simulink model "abs"  (R2023b)
settings: Solver=VariableStepAuto  StartTime=0.0  StopTime=25  RelTol=1e-3
undefined symbols (not defined in the file): g, I, m, muCoefficientOfFriction, R, Slip, v0
settings Model: Creator=Asus  LastModifiedBy=Asus

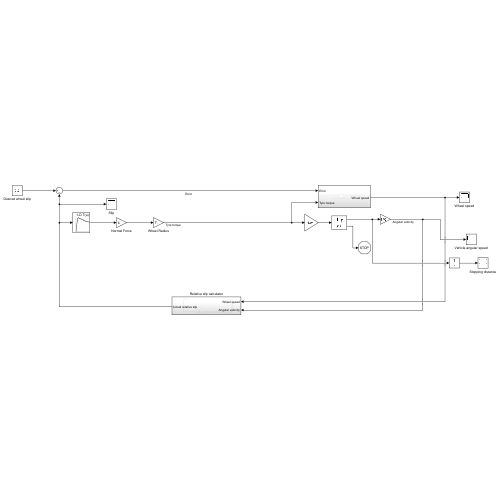
[thumbnail: Simulink's stored preview of the top-level diagram]
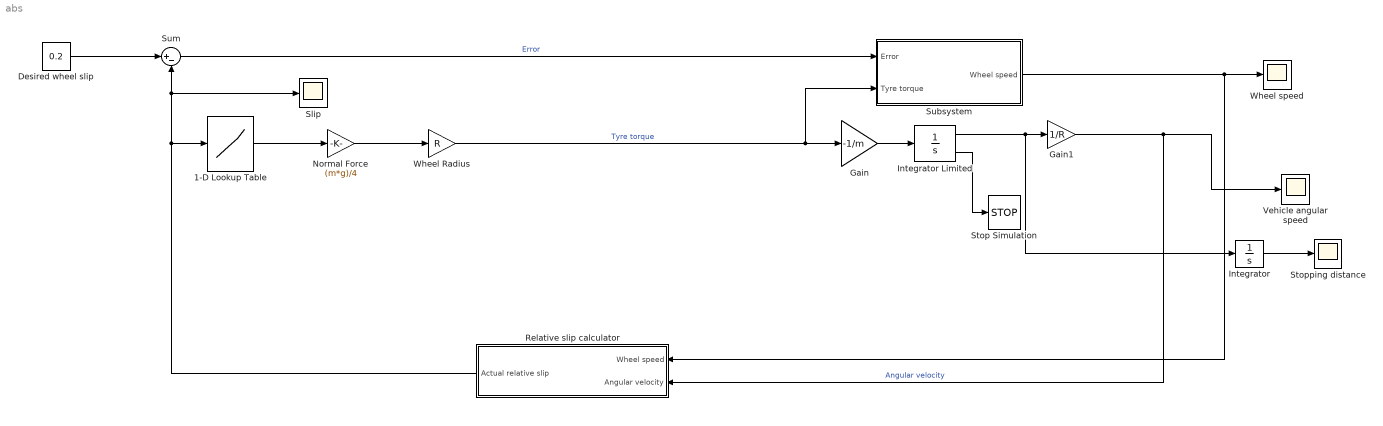
== system abs ==
  1-D Lookup Table : Lookup_n-D  NumberOfTableDimensions=1  BreakpointsForDimension1=muCoefficientOfFriction  Table=Slip  InternalRulePriority=Speed  RndMeth=Simplest
  Desired wheel slip : Constant  Value=0.2  SampleTime=-1
  Gain : Gain  Gain=-1/m
  Gain1 : Gain  Gain=1/R
  Integrator : Integrator
  Integrator Limited : Integrator  InitialCondition=v0  LimitOutput=on  UpperSaturationLimit=1000  LowerSaturationLimit=0  ShowSaturationPort=on
  Normal Force : Gain  Gain=(m*g)/4
  Relative slip calculator : Subsystem
  Slip : Scope
  Stop Simulation : Stop
  Stopping distance : Scope
  Subsystem : Subsystem
  Sum : Sum  Inputs=|+-
  Vehicle angular speed : Scope
  Wheel Radius : Gain  Gain=R
  Wheel speed : Scope
  wires:
  Desired wheel slip/1 -> Sum/1
  1-D Lookup Table/1 -> Normal Force/1
  Normal Force/1 -> Wheel Radius/1
  Sum/1 -> Subsystem/1(Error)  "Error"
  Wheel Radius/1 -> Gain/1, Subsystem/2(Tyre torque)  "Tyre torque"
  Subsystem/1(Wheel speed) -> Wheel speed/1, Relative slip calculator/1(Wheel speed)
  Gain/1 -> Integrator Limited/1
  Integrator Limited/2 -> Stop Simulation/1
  Integrator Limited/1 -> Integrator/1, Gain1/1
  Gain1/1 -> Relative slip calculator/2(Angular velocity), Vehicle angular speed/1  "Angular velocity"
  Integrator/1 -> Stopping distance/1
  Relative slip calculator/1(Actual relative slip) -> 1-D Lookup Table/1, Slip/1, Sum/2

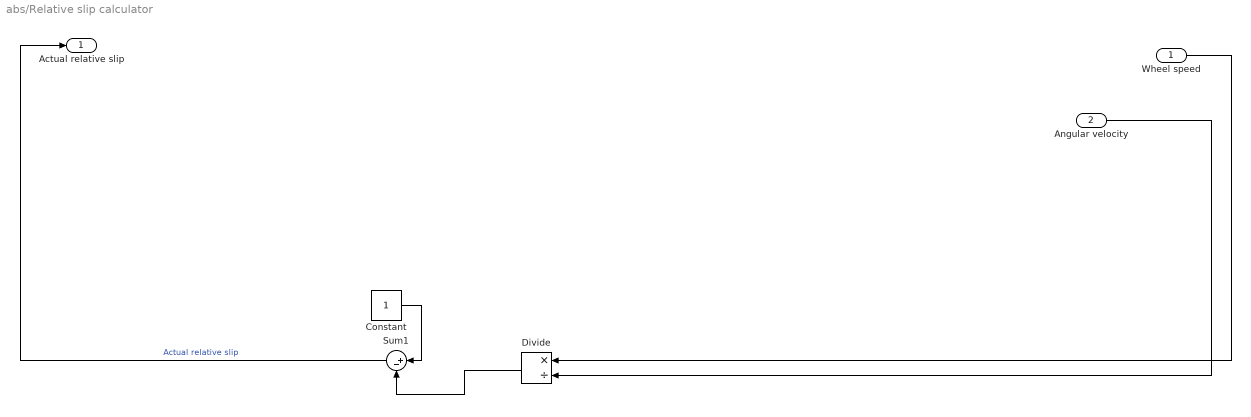
== system abs/Relative slip calculator ==
  Wheel speed : Inport
  Angular velocity : Inport  Port=2
  Constant : Constant
  Divide : Product  Inputs=*/
  Sum1 : Sum  Inputs=|+-
  Actual relative slip : Outport
  wires:
  Constant/1 -> Sum1/1
  Divide/1 -> Sum1/2
  Angular velocity/1 -> Divide/2
  Sum1/1 -> Actual relative slip/1  "Actual relative slip"
  Wheel speed/1 -> Divide/1

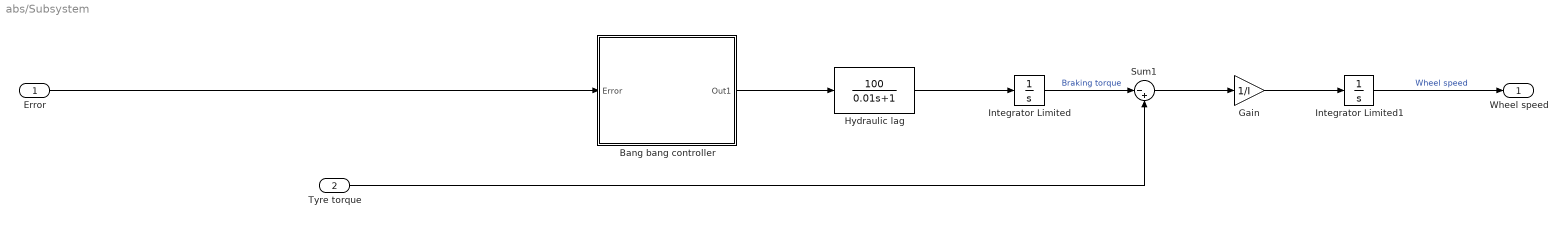
== system abs/Subsystem ==
  Error : Inport
  Tyre torque : Inport  Port=2
  Bang bang controller : Subsystem
  Gain : Gain  Gain=1/I
  Hydraulic lag : TransferFcn  Numerator=[100]  Denominator=[0.01 1]
  Integrator Limited : Integrator  LimitOutput=on  UpperSaturationLimit=1000  LowerSaturationLimit=0
  Integrator Limited1 : Integrator  InitialCondition=v0/R  LimitOutput=on  UpperSaturationLimit=1000  LowerSaturationLimit=0
  Sum1 : Sum  Inputs=|-+
  Wheel speed : Outport
  wires:
  Sum1/1 -> Gain/1
  Integrator Limited/1 -> Sum1/1  "Braking torque"
  Gain/1 -> Integrator Limited1/1
  Bang bang controller/1(Out1) -> Hydraulic lag/1
  Integrator Limited1/1 -> Wheel speed/1  "Wheel speed"
  Hydraulic lag/1 -> Integrator Limited/1
  Error/1 -> Bang bang controller/1(Error)
  Tyre torque/1 -> Sum1/2

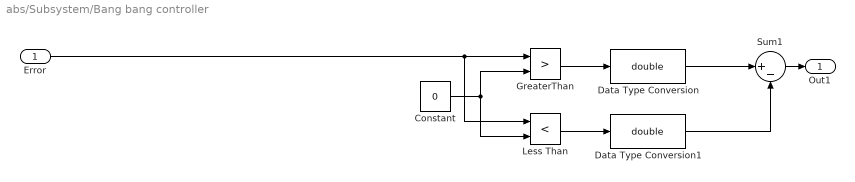
== system abs/Subsystem/Bang bang controller ==
  Error : Inport
  Constant : Constant  Value=0
  Data Type Conversion : DataTypeConversion  OutDataTypeStr=double  SaturateOnIntegerOverflow=off
  Data Type Conversion1 : DataTypeConversion  OutDataTypeStr=double  SaturateOnIntegerOverflow=off
  GreaterThan : RelationalOperator  Operator=>  OutDataTypeStr=boolean  RndMeth=Simplest  InputSameDT=off
  Less Than : RelationalOperator  Operator=<  OutDataTypeStr=boolean  RndMeth=Simplest  InputSameDT=off
  Sum1 : Sum  Inputs=|+-
  Out1 : Outport
  wires:
  Data Type Conversion/1 -> Sum1/1
  Less Than/1 -> Data Type Conversion1/1
  Data Type Conversion1/1 -> Sum1/2
  Constant/1 -> Less Than/2, GreaterThan/2
  Error/1 -> Less Than/1, GreaterThan/1
  GreaterThan/1 -> Data Type Conversion/1
  Sum1/1 -> Out1/1
